simulink model "Tricopter_Controlled"  (R2015a)
settings: Solver=ode3  SolverMode=SingleTasking  StartTime=0.0  StopTime=inf  FixedStep=T_sim  RelTol=1e-3
values from neighbouring files (symbols this model uses):
  A_l_max_x = sqrt( (A_z_max)^2  -  g^2  )    [Run3Copter.m]
  A_l_max_y = g*tand(15)    [Run3Copter.m]
  A_z_max = Max_Thrust*3/m    [Run3Copter.m]
  Alt_0 = input(' Give the initial altitude (m): ')    [Run3Copter.m]
  B_hover_4dof = [-0.192641491537 -0.295051706147 -72.3190840892 -0.00308714144823 24.9504828653 -1.18743631629 9.87469464114e-05 6.48783896558 -0.0529805907426 -0.000387203135788 0.131620058452 2.24065603044 ... (54 elements, 6x9)]    [Effectiv_matrices.mat]
  CG_0 = [0,0,0.02]'    [SetupComplete.m]
  epsilon = 0.01    [Run3Copter.m]
  eta_23 = deg2rad(-1.3)    [Run3Copter.m]
  g = 9.81    [SetupComplete.m]
  h = 0.08    [SetupComplete.m]
  h_M = 0.064    [SetupComplete.m]
  Hover_eta_23 = deg2rad(-1.3)    [Run3Copter.m]
  Hover_throtle_1 = 0.745    [Run3Copter.m]
  Hover_throtle_23 = Hover_throtle_1/cos(Hover_eta_23)    [Run3Copter.m]
  I_BAC_0 = [ Ix,0,Ixz;0,Iy,0;Ixz,0,Iz]    [SetupComplete.m]
  Initial_Omegas = Omega_hover    [Run3Copter.m]
  Initial_Torques = Torque_hover    [Run3Copter.m]
  Ix = 0.103    [SetupComplete.m]
  Iy = 0.147    [SetupComplete.m]
  Iz = 0.237    [SetupComplete.m]
  l = 0.345    [SetupComplete.m]
  l_arm = 0.264    [SetupComplete.m]
  latitude = 52.071118    [Run3Copter.m]
  longitude = -0.627404    [Run3Copter.m]
  m = 3.51    [SetupComplete.m]
  m_0 = 2.61    [SetupComplete.m]
  m_M = 0.300    (= 0.3)    [SetupComplete.m]
  Rotation_sign = [ 1,-1,-1]    [SetupComplete.m]
  T_ctrl = 0.02    [Run3Copter.m]
  T_sim = 0.01    [Run3Copter.m]
  throtle_1 = 0*0.745    (= 0)    [Run3Copter.m]
  throtle_23 = throtle_1/cos(eta_23)    [Run3Copter.m]
  v_i0 = sqrt( 1/3*m*g/(2*rho*pi*R^2)  )    [SetupComplete.m]
undefined symbols (not defined in the file or in its folder): DOWN_0, EAST_0, Newton, NORTH_0, P_0, Q_0, R_0, Raphson, U_0, V_0, W_0
libraries: XXCopter_Control x64, simulink_extras x17, simulink x11, XXCopter x8
(part 5 of 6)

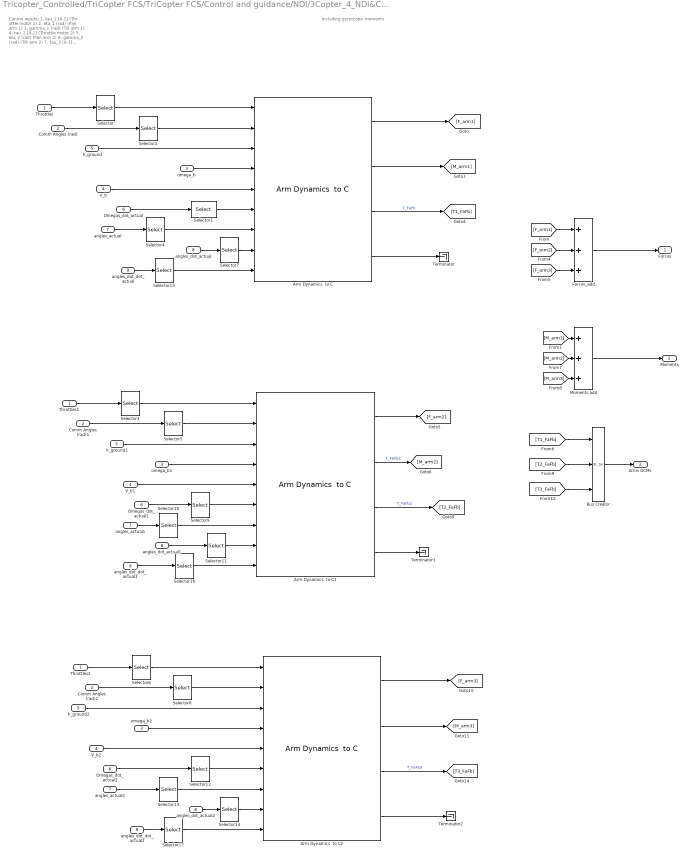
== system Tricopter_Controlled/TriCopter FCS/TriCopter FCS/Control and guidance/NDI/3Copter_4_NDI&CA/Arms Dynamics: Forces and Moments ==
  note: Including gyroscopic moments
  note: Control inputs:
      | 1. tau_1 [0-1] (Thr ottle motor 1)
      | 2. eta_1 (rad)  (Pan arm 1)
      | 3. gamma_1 (rad)  (Tilt arm 1)
      |
      | 4. tau_2 [0-1] (Throttle motor 2)
      | 5. eta_2 (rad)  (Pan arm 2)
      | 6. gamma_2 (rad)  (Tilt arm 2)
      |
      | 7. tau_3 [0-1] (Throttle motor 3)
      | 8. eta_3 (rad)  (Pan arm  3)
      | 9. gamma_3 (rad)  (Tilt arm 3)
  Throttles : Inport
  Comm Angles (rad) : Inport  Port=2
  omega_b : Inport  Port=3
  V_b : Inport  Port=4
  h_ground : Inport  Port=5
  Omegas_dot_actual : Inport  Port=6
  angles_actual : Inport  Port=7
  angles_dot_actual : Inport  Port=8
  angles_dot_dot_actual : Inport  Port=9
  Arm Dynamics  to C : XXCopter_Control/Arm Dynamics  to C  Rot_sign=Rotation_sign(1)  arm_hub_pos=l*[1;0;0]  Arm_axis=[l_arm;0;0]  arm_num=1  eta_dir=[1;0;0]  gamma_dir=[0;1;0]  J_T=J_T  J_FA=J_FA  h=h  switch_val=direct_feedforward  omega_n=30  xi=1.4  eta_inf_lim=deg2rad(-180)  eta_sup_lim=deg2rad(180)  gamma_inf_lim=deg2rad(-90)  gamma_sup_lim=deg2rad(15)
  Arm Dynamics  to C1 : XXCopter_Control/Arm Dynamics  to C  Rot_sign=Rotation_sign(2)  arm_hub_pos=l*[-1/2;sqrt(3)/2;0]  Arm_axis=[0;l_arm;0]  arm_num=2  eta_dir=[0;1;0]  gamma_dir=[1;0;0]  J_T=J_T  J_FA=J_FA  h=h  switch_val=direct_feedforward  omega_n=30  xi=1.4  eta_inf_lim=deg2rad(-180)  eta_sup_lim=deg2rad(180)  gamma_inf_lim=deg2rad(-15)  gamma_sup_lim=deg2rad(90)
  Arm Dynamics  to C2 : XXCopter_Control/Arm Dynamics  to C  Rot_sign=Rotation_sign(3)  arm_hub_pos=l*[-1/2;-sqrt(3)/2;0]  Arm_axis=[0;-l_arm;0]  arm_num=3  eta_dir=[0;1;0]  gamma_dir=[1;0;0]  J_T=J_T  J_FA=J_FA  h=h  switch_val=direct_feedforward  omega_n=30  xi=1.4  eta_inf_lim=deg2rad(-180)  eta_sup_lim=deg2rad(180)  gamma_inf_lim=deg2rad(-90)  gamma_sup_lim=deg2rad(15)
  Bus Creator : BusCreator  Inputs=3
  Comm Angles (rad)1 : InportShadow  Port=2
  Comm Angles (rad)2 : InportShadow  Port=2
  Forces_add : Sum  Inputs=+++
  Moments add : Sum  Inputs=+++
  Omegas_dot_actual1 : InportShadow  Port=6
  Omegas_dot_actual2 : InportShadow  Port=6
  Selector : Selector  IndexMode=Zero-based  InputPortWidth=3  Indices=0
  Selector1 : Selector  IndexMode=Zero-based  InputPortWidth=3  Indices=0
  Selector{5,10..11,16} (4 alike) : Selector  IndexMode=Zero-based  InputPortWidth=6  Indices=[2,3]
  Selector12 : Selector  IndexMode=Zero-based  InputPortWidth=3  Indices=2
  Selector{8,13..14,17} (4 alike) : Selector  IndexMode=Zero-based  InputPortWidth=6  Indices=[4,5]
  Selector{2,4,7,15} (4 alike) : Selector  IndexMode=Zero-based  InputPortWidth=6  Indices=[0,1]
  Selector3 : Selector  IndexMode=Zero-based  InputPortWidth=3
  Selector6 : Selector  IndexMode=Zero-based  InputPortWidth=3  Indices=2
  Selector9 : Selector  IndexMode=Zero-based  InputPortWidth=3
  Terminator : Terminator
  Terminator1 : Terminator
  Terminator2 : Terminator
  Throttles1 : InportShadow
  Throttles2 : InportShadow
  V_b1 : InportShadow  Port=4
  V_b2 : InportShadow  Port=4
  angles_actual1 : InportShadow  Port=7
  angles_actual2 : InportShadow  Port=7
  angles_dot_actual1 : InportShadow  Port=8
  angles_dot_actual2 : InportShadow  Port=8
  angles_dot_dot_actual1 : InportShadow  Port=9
  angles_dot_dot_actual2 : InportShadow  Port=9
  h_ground1 : InportShadow  Port=5
  h_ground2 : InportShadow  Port=5
  omega_b1 : InportShadow  Port=3
  omega_b2 : InportShadow  Port=3
  Forces : Outport
  Moments : Outport  Port=2
  Arms DCMs : Outport  Port=3
  wires:
  Selector14/1 -> Arm Dynamics  to C2/8
  angles_actual2/1 -> Selector13/1
  angles_dot_actual2/1 -> Selector14/1
  Selector13/1 -> Arm Dynamics  to C2/7
  Selector12/1 -> Arm Dynamics  to C2/6
  Omegas_dot_actual2/1 -> Selector12/1
  Selector11/1 -> Arm Dynamics  to C1/8
  angles_actual1/1 -> Selector10/1
  angles_dot_actual1/1 -> Selector11/1
  Selector10/1 -> Arm Dynamics  to C1/7
  Selector9/1 -> Arm Dynamics  to C1/6
  Omegas_dot_actual1/1 -> Selector9/1
  Selector7/1 -> Arm Dynamics  to C/8
  angles_dot_actual/1 -> Selector7/1
  Selector4/1 -> Arm Dynamics  to C/7
  angles_actual/1 -> Selector4/1
  Selector1/1 -> Arm Dynamics  to C/6
  Omegas_dot_actual/1 -> Selector1/1
  [T3_FaFb] -> Bus Creator/3
  [T2_FaFb] -> Bus Creator/2
  [T1_FaFb] -> Bus Creator/1
  Bus Creator/1 -> Arms DCMs/1
  Arm Dynamics  to C1/2 -> [M_arm2]  "T_FaFb2"
  Arm Dynamics  to C1/1 -> [F_arm2]
  Arm Dynamics  to C2/4 -> Terminator2/1
  Arm Dynamics  to C1/4 -> Terminator1/1
  Arm Dynamics  to C/4 -> Terminator/1
  Arm Dynamics  to C2/3 -> [T3_FaFb]  "T_FaFb3"
  Comm Angles (rad)2/1 -> Selector8/1
  Selector8/1 -> Arm Dynamics  to C2/2
  omega_b2/1 -> Arm Dynamics  to C2/4
  Arm Dynamics  to C2/2 -> [M_arm3]
  Arm Dynamics  to C2/1 -> [F_arm3]
  h_ground2/1 -> Arm Dynamics  to C2/3
  V_b2/1 -> Arm Dynamics  to C2/5
  Selector6/1 -> Arm Dynamics  to C2/1
  Throttles2/1 -> Selector6/1
  Arm Dynamics  to C1/3 -> [T2_FaFb]  "T_FaFb2"
  Comm Angles (rad)1/1 -> Selector5/1
  Selector5/1 -> Arm Dynamics  to C1/2
  omega_b1/1 -> Arm Dynamics  to C1/4
  h_ground1/1 -> Arm Dynamics  to C1/3
  V_b1/1 -> Arm Dynamics  to C1/5
  Selector3/1 -> Arm Dynamics  to C1/1
  Throttles1/1 -> Selector3/1
  Arm Dynamics  to C/3 -> [T1_FaFb]  "T_FaFb"
  Comm Angles (rad)/1 -> Selector2/1
  Selector2/1 -> Arm Dynamics  to C/2
  [M_arm2] -> Moments add/2
  [M_arm3] -> Moments add/3
  [F_arm3] -> Forces_add/3
  [F_arm2] -> Forces_add/2
  omega_b/1 -> Arm Dynamics  to C/4
  [M_arm1] -> Moments add/1
  [F_arm1] -> Forces_add/1
  Arm Dynamics  to C/2 -> [M_arm1]
  Arm Dynamics  to C/1 -> [F_arm1]
  h_ground/1 -> Arm Dynamics  to C/3
  Moments add/1 -> Moments/1
  Forces_add/1 -> Forces/1
  V_b/1 -> Arm Dynamics  to C/5
  Selector/1 -> Arm Dynamics  to C/1
  Throttles/1 -> Selector/1
  angles_dot_dot_actual/1 -> Selector15/1
  Selector15/1 -> Arm Dynamics  to C/9
  angles_dot_dot_actual1/1 -> Selector16/1
  Selector16/1 -> Arm Dynamics  to C1/9
  angles_dot_dot_actual2/1 -> Selector17/1
  Selector17/1 -> Arm Dynamics  to C2/9

== system Tricopter_Controlled/TriCopter FCS/TriCopter FCS/Control and guidance/NDI/3Copter_4_NDI&CA/Gradient ==
  note: Control inputs:
      | 1. tau_1 [0-1] (Thr ottle motor 1)
      | 2. eta_1 (rad)  (Pan arm 1)
      | 3. gamma_1 (rad)  (Tilt arm 1)
      |
      | 4. tau_2 [0-1] (Throttle motor 2)
      | 5. eta_2 (rad)  (Pan arm 2)
      | 6. gamma_2 (rad)  (Tilt arm 2)
      |
      | 7. tau_3 [0-1] (Throttle motor 3)
      | 8. eta_3 (rad)  (Pan arm  3)
      | 9. gamma_3 (rad)  (Tilt arm 3)
  Curr_V : Inport  Partition=off
  "Control Inputs(rad) " : Inport  Port=2  Partition=on  PartitionDimension=1  PartitionWidth=9
  h : Inport  Port=3  Partition=off
  Vb : Inport  Port=4  Partition=off
  omega_b : Inport  Port=5  Partition=off
  Omegas_dot_actual : Inport  Port=6  Partition=off
  angles_actual : Inport  Port=7  Partition=off
  angles_dot_actual : Inport  Port=8  Partition=off
  angles_dot_dot_actual : Inport  Port=9  Partition=off
  F_g : Inport  Port=10  Partition=off
  M_g : Inport  Port=11  Partition=off
  Add : Sum
  Add1 : Sum
  Arms Dynamics: Forces and Moments : Subsystem  TreatAsAtomicUnit=on
  Equivalent Throttle : Product  Inputs=**
  For Each : ForEach  DisableCoverage=on  IndexMode=One-based
  Mux : Mux  Inputs=[3,3]
  Signal Specification : SignalSpecification  Dimensions=[6,1]
  Terminator : Terminator
  Throttles : Selector  IndexMode=Zero-based  InputPortWidth=9  Indices=[0,3,6]
  "angles " : Selector  IndexMode=Zero-based  InputPortWidth=9  Indices=[1,2,4,5,7,8]
  Forces_Moments : Outport  ConcatenationDimension=2
  wires:
  Signal Specification/1 -> Forces_Moments/1
  Mux/1 -> Signal Specification/1
  Add1/1 -> Mux/2
  Add/1 -> Mux/1
  M_g/1 -> Add1/2
  F_g/1 -> Add/2
  angles_dot_actual/1 -> Arms Dynamics: Forces and Moments/8(angles_dot_actual)
  Omegas_dot_actual/1 -> Arms Dynamics: Forces and Moments/6(Omegas_dot_actual)
  Curr_V/1 -> Equivalent Throttle/1
  Equivalent Throttle/1 -> Arms Dynamics: Forces and Moments/1(Throttles)
  "Control Inputs(rad) "/1 -> "angles "/1, Throttles/1
  Throttles/1 -> Equivalent Throttle/2
  Arms Dynamics: Forces and Moments/1(Forces) -> Add/1
  h/1 -> Arms Dynamics: Forces and Moments/5(h_ground)
  omega_b/1 -> Arms Dynamics: Forces and Moments/3(omega_b)
  angles_actual/1 -> Arms Dynamics: Forces and Moments/7(angles_actual)
  "angles "/1 -> Arms Dynamics: Forces and Moments/2(Comm Angles (rad))
  angles_dot_dot_actual/1 -> Arms Dynamics: Forces and Moments/9(angles_dot_dot_actual)
  Arms Dynamics: Forces and Moments/2(Moments) -> Add1/1
  Arms Dynamics: Forces and Moments/3(Arms DCMs) -> Terminator/1
  Vb/1 -> Arms Dynamics: Forces and Moments/4(V_b)

== system Tricopter_Controlled/TriCopter FCS/TriCopter FCS/Control and guidance/NDI/3Copter_4_NDI&CA/Ground  model ==
  h : Inport
  m : Inport  Port=2
  q : Inport  Port=3
  Ground model logic and Forces and moments : MATLAB Function  TreatAsAtomicUnit=on
  arm_hub position 1 : Constant  Value=l*[1;0;0]
  arm_hub position 2 : Constant  Value=l*[-1/2;sqrt(3)/2;0]
  arm_hub position 3 : Constant  Value=l*[-1/2;-sqrt(3)/2;0]
  F_ground : Outport
  wires:
  h/1 -> Ground model logic and Forces and moments/1(h)
  m/1 -> Ground model logic and Forces and moments/2(mass)
  arm_hub position 1/1 -> Ground model logic and Forces and moments/4(Arm1)
  arm_hub position 2/1 -> Ground model logic and Forces and moments/5(Arm2)
  arm_hub position 3/1 -> Ground model logic and Forces and moments/6(Arm3)
  Ground model logic and Forces and moments/1(F_gr_b) -> F_ground/1
  q/1 -> Ground model logic and Forces and moments/3(q)

== system Tricopter_Controlled/TriCopter FCS/TriCopter FCS/Control and guidance/NDI/3Copter_4_NDI&CA/Mass Properties ==
  Arms DCMs : Inport
  CG_0 : Inport  Port=2
  m_0 : Inport  Port=3
  m : Inport  Port=4
  m_M : Inport  Port=5
  I_BAC_0 : Inport  Port=6
  Arm Inertia : MATLAB Function  TreatAsAtomicUnit=on
  Bus Selector : BusSelector  OutputSignals=T_FaFb,T_FaFb2,T_FaFb3
  CG position : Sum
  Divide : Product  Inputs=*/
  Divide1 : Product  Inputs=**
  Divide2 : Product  Inputs=/*
  Divide3 : Product  Inputs=**
  Motors Pos sum : Sum  Inputs=+++
  Total I_BAC : Sum
  I_BAC : Outport
  CG : Outport  Port=2
  wires:
  Arm Inertia/2(r1_M) -> Motors Pos sum/3
  I_BAC_0/1 -> Total I_BAC/1
  Arm Inertia/1(I_M) -> Total I_BAC/2
  Arm Inertia/4(r3_M) -> Motors Pos sum/1
  Arm Inertia/3(r2_M) -> Motors Pos sum/2
  Divide3/1 -> CG position/2
  Divide2/1 -> Divide3/2
  Motors Pos sum/1 -> Divide3/1
  Divide1/1 -> CG position/1
  CG position/1 -> CG/1
  m_M/1 -> Divide2/2
  Divide/1 -> Divide1/2
  CG_0/1 -> Divide1/1
  m/1 -> Divide2/1, Divide/2
  m_0/1 -> Divide/1
  Total I_BAC/1 -> I_BAC/1
  Bus Selector/1 -> Arm Inertia/1(T1_FAFb)  "<T_FaFb>"
  Bus Selector/2 -> Arm Inertia/2(T2_FAFb)  "<T_FaFb2>"
  Bus Selector/3 -> Arm Inertia/3(T3_FAFb)  "<T_FaFb3>"
  Arms DCMs/1 -> Bus Selector/1

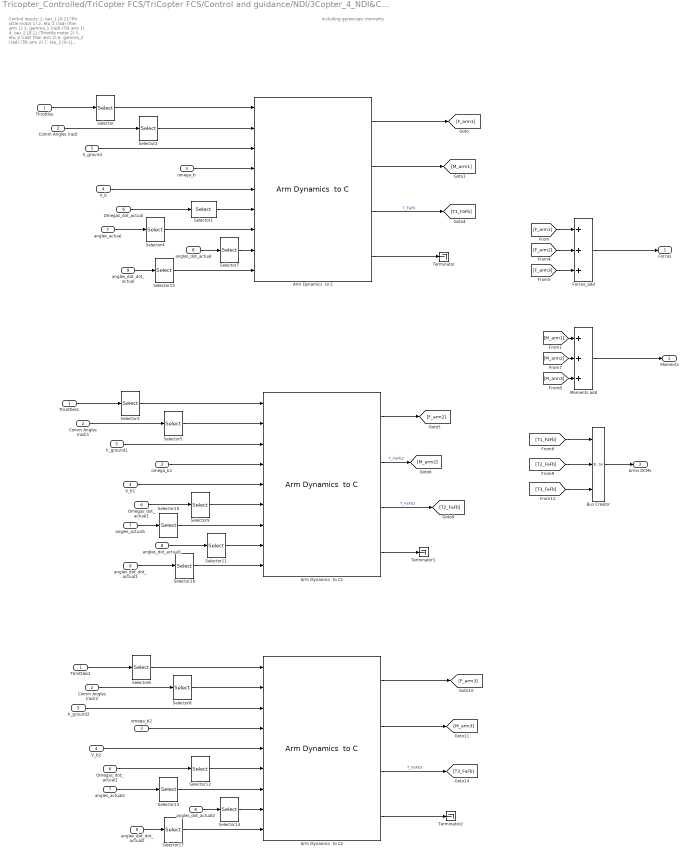
== system Tricopter_Controlled/TriCopter FCS/TriCopter FCS/Control and guidance/NDI/3Copter_4_NDI&CA/Gradient/Arms Dynamics: Forces and Moments ==
  note: Including gyroscopic moments
  note: Control inputs:
      | 1. tau_1 [0-1] (Thr ottle motor 1)
      | 2. eta_1 (rad)  (Pan arm 1)
      | 3. gamma_1 (rad)  (Tilt arm 1)
      |
      | 4. tau_2 [0-1] (Throttle motor 2)
      | 5. eta_2 (rad)  (Pan arm 2)
      | 6. gamma_2 (rad)  (Tilt arm 2)
      |
      | 7. tau_3 [0-1] (Throttle motor 3)
      | 8. eta_3 (rad)  (Pan arm  3)
      | 9. gamma_3 (rad)  (Tilt arm 3)
  Throttles : Inport
  Comm Angles (rad) : Inport  Port=2
  omega_b : Inport  Port=3
  V_b : Inport  Port=4
  h_ground : Inport  Port=5
  Omegas_dot_actual : Inport  Port=6
  angles_actual : Inport  Port=7
  angles_dot_actual : Inport  Port=8
  angles_dot_dot_actual : Inport  Port=9
  Arm Dynamics  to C : XXCopter_Control/Arm Dynamics  to C  Rot_sign=Rotation_sign(1)  arm_hub_pos=l*[1;0;0]  Arm_axis=[l_arm;0;0]  arm_num=1  eta_dir=[1;0;0]  gamma_dir=[0;1;0]  J_T=J_T  J_FA=J_FA  h=h  switch_val=direct_feedforward  omega_n=30  xi=1.4  eta_inf_lim=deg2rad(-180)  eta_sup_lim=deg2rad(180)  gamma_inf_lim=deg2rad(-90)  gamma_sup_lim=deg2rad(15)
  Arm Dynamics  to C1 : XXCopter_Control/Arm Dynamics  to C  Rot_sign=Rotation_sign(2)  arm_hub_pos=l*[-1/2;sqrt(3)/2;0]  Arm_axis=[0;l_arm;0]  arm_num=2  eta_dir=[0;1;0]  gamma_dir=[1;0;0]  J_T=J_T  J_FA=J_FA  h=h  switch_val=direct_feedforward  omega_n=30  xi=1.4  eta_inf_lim=deg2rad(-180)  eta_sup_lim=deg2rad(180)  gamma_inf_lim=deg2rad(-15)  gamma_sup_lim=deg2rad(90)
  Arm Dynamics  to C2 : XXCopter_Control/Arm Dynamics  to C  Rot_sign=Rotation_sign(3)  arm_hub_pos=l*[-1/2;-sqrt(3)/2;0]  Arm_axis=[0;-l_arm;0]  arm_num=3  eta_dir=[0;1;0]  gamma_dir=[1;0;0]  J_T=J_T  J_FA=J_FA  h=h  switch_val=direct_feedforward  omega_n=30  xi=1.4  eta_inf_lim=deg2rad(-180)  eta_sup_lim=deg2rad(180)  gamma_inf_lim=deg2rad(-90)  gamma_sup_lim=deg2rad(15)
  Bus Creator : BusCreator  Inputs=3
  Comm Angles (rad)1 : InportShadow  Port=2
  Comm Angles (rad)2 : InportShadow  Port=2
  Forces_add : Sum  Inputs=+++
  Moments add : Sum  Inputs=+++
  Omegas_dot_actual1 : InportShadow  Port=6
  Omegas_dot_actual2 : InportShadow  Port=6
  Selector : Selector  IndexMode=Zero-based  InputPortWidth=3  Indices=0
  Selector1 : Selector  IndexMode=Zero-based  InputPortWidth=3  Indices=0
  Selector{5,10..11,16} (4 alike) : Selector  IndexMode=Zero-based  InputPortWidth=6  Indices=[2,3]
  Selector12 : Selector  IndexMode=Zero-based  InputPortWidth=3  Indices=2
  Selector{8,13..14,17} (4 alike) : Selector  IndexMode=Zero-based  InputPortWidth=6  Indices=[4,5]
  Selector{2,4,7,15} (4 alike) : Selector  IndexMode=Zero-based  InputPortWidth=6  Indices=[0,1]
  Selector3 : Selector  IndexMode=Zero-based  InputPortWidth=3
  Selector6 : Selector  IndexMode=Zero-based  InputPortWidth=3  Indices=2
  Selector9 : Selector  IndexMode=Zero-based  InputPortWidth=3
  Terminator : Terminator
  Terminator1 : Terminator
  Terminator2 : Terminator
  Throttles1 : InportShadow
  Throttles2 : InportShadow
  V_b1 : InportShadow  Port=4
  V_b2 : InportShadow  Port=4
  angles_actual1 : InportShadow  Port=7
  angles_actual2 : InportShadow  Port=7
  angles_dot_actual1 : InportShadow  Port=8
  angles_dot_actual2 : InportShadow  Port=8
  angles_dot_dot_actual1 : InportShadow  Port=9
  angles_dot_dot_actual2 : InportShadow  Port=9
  h_ground1 : InportShadow  Port=5
  h_ground2 : InportShadow  Port=5
  omega_b1 : InportShadow  Port=3
  omega_b2 : InportShadow  Port=3
  Forces : Outport
  Moments : Outport  Port=2
  Arms DCMs : Outport  Port=3
  wires:
  Selector14/1 -> Arm Dynamics  to C2/8
  angles_actual2/1 -> Selector13/1
  angles_dot_actual2/1 -> Selector14/1
  Selector13/1 -> Arm Dynamics  to C2/7
  Selector12/1 -> Arm Dynamics  to C2/6
  Omegas_dot_actual2/1 -> Selector12/1
  Selector11/1 -> Arm Dynamics  to C1/8
  angles_actual1/1 -> Selector10/1
  angles_dot_actual1/1 -> Selector11/1
  Selector10/1 -> Arm Dynamics  to C1/7
  Selector9/1 -> Arm Dynamics  to C1/6
  Omegas_dot_actual1/1 -> Selector9/1
  Selector7/1 -> Arm Dynamics  to C/8
  angles_dot_actual/1 -> Selector7/1
  Selector4/1 -> Arm Dynamics  to C/7
  angles_actual/1 -> Selector4/1
  Selector1/1 -> Arm Dynamics  to C/6
  Omegas_dot_actual/1 -> Selector1/1
  [T3_FaFb] -> Bus Creator/3
  [T2_FaFb] -> Bus Creator/2
  [T1_FaFb] -> Bus Creator/1
  Bus Creator/1 -> Arms DCMs/1
  Arm Dynamics  to C1/2 -> [M_arm2]  "T_FaFb2"
  Arm Dynamics  to C1/1 -> [F_arm2]
  Arm Dynamics  to C2/4 -> Terminator2/1
  Arm Dynamics  to C1/4 -> Terminator1/1
  Arm Dynamics  to C/4 -> Terminator/1
  Arm Dynamics  to C2/3 -> [T3_FaFb]  "T_FaFb3"
  Comm Angles (rad)2/1 -> Selector8/1
  Selector8/1 -> Arm Dynamics  to C2/2
  omega_b2/1 -> Arm Dynamics  to C2/4
  Arm Dynamics  to C2/2 -> [M_arm3]
  Arm Dynamics  to C2/1 -> [F_arm3]
  h_ground2/1 -> Arm Dynamics  to C2/3
  V_b2/1 -> Arm Dynamics  to C2/5
  Selector6/1 -> Arm Dynamics  to C2/1
  Throttles2/1 -> Selector6/1
  Arm Dynamics  to C1/3 -> [T2_FaFb]  "T_FaFb2"
  Comm Angles (rad)1/1 -> Selector5/1
  Selector5/1 -> Arm Dynamics  to C1/2
  omega_b1/1 -> Arm Dynamics  to C1/4
  h_ground1/1 -> Arm Dynamics  to C1/3
  V_b1/1 -> Arm Dynamics  to C1/5
  Selector3/1 -> Arm Dynamics  to C1/1
  Throttles1/1 -> Selector3/1
  Arm Dynamics  to C/3 -> [T1_FaFb]  "T_FaFb"
  Comm Angles (rad)/1 -> Selector2/1
  Selector2/1 -> Arm Dynamics  to C/2
  [M_arm2] -> Moments add/2
  [M_arm3] -> Moments add/3
  [F_arm3] -> Forces_add/3
  [F_arm2] -> Forces_add/2
  omega_b/1 -> Arm Dynamics  to C/4
  [M_arm1] -> Moments add/1
  [F_arm1] -> Forces_add/1
  Arm Dynamics  to C/2 -> [M_arm1]
  Arm Dynamics  to C/1 -> [F_arm1]
  h_ground/1 -> Arm Dynamics  to C/3
  Moments add/1 -> Moments/1
  Forces_add/1 -> Forces/1
  V_b/1 -> Arm Dynamics  to C/5
  Selector/1 -> Arm Dynamics  to C/1
  Throttles/1 -> Selector/1
  angles_dot_dot_actual/1 -> Selector15/1
  Selector15/1 -> Arm Dynamics  to C/9
  angles_dot_dot_actual1/1 -> Selector16/1
  Selector16/1 -> Arm Dynamics  to C1/9
  angles_dot_dot_actual2/1 -> Selector17/1
  Selector17/1 -> Arm Dynamics  to C2/9

== matlab function Tricopter_Controlled/3 Copter Complete/6dof Eqs of motion/Position Eqs ==
  data: A_b output; Vb input; omega input; omega_dot input; Forces input; m input; CG input
function A_b  = PositionEqs(Vb,omega,omega_dot, Forces,m, CG)



 
A_b =  1/m*( Forces ) - cross(omega,Vb) - cross(omega, cross(omega,CG)) -cross(omega_dot,CG)  ;

== matlab function Tricopter_Controlled/3 Copter Complete/6dof Eqs of motion/Rotational eqs ==
  data: omega_dot output; omega_b input; Moments input; I_BAC input
function omega_dot  = Rotational_Eq(omega_b,Moments, I_BAC)



omega_dot =  I_BAC\( Moments - cross(omega_b,I_BAC*omega_b)  );

== matlab function Tricopter_Controlled/3 Copter Complete/6dof Eqs of motion/q_dot/Quaternion_dot ==
  data: omega_b input; q_dot output; q input
function q_dot = Quaternion_dot(omega_b,q)


q_dot = 1/2*HamiltonProduct(q,[0;omega_b]);

function Product= HamiltonProduct( a,b )

Product=[ a(1)*b(1)-a(2)*b(2)-a(3)*b(3)-a(4)*b(4) ; a(1)*b(2)+a(2)*b(1)+a(3)*b(4)-a(4)*b(3)  ; a(1)*b(3)-a(2)*b(4)+a(3)*b(1)+a(4)*b(2)  ; a(1)*b(4)+a(2)*b(3)-a(3)*b(2)+a(4)*b(1) ];

== matlab function Tricopter_Controlled/TriCopter FCS/TriCopter FCS/Flight mode manager and commands generator/Flight manager/Parameters_based_decision_making ==
  data: flight_mode_out output; flight_mode input; pdop input; vdop input; num_sats input; Alt input; Volt input; Accs input
function flight_mode_out     =  Params_decision_making(flight_mode,pdop,vdop,num_sats,Alt,Volt,Accs)

% si esta en landing y recive una aceleracion vertical de <-5m/s^2( Hacia
% arriba), pasar a modo OFF

% If ready from off blue LED
flight_mode_out = flight_mode;
 switch flight_mode % Being in this FM
        case 0 % Off
           
        case 1 % Ready
         
        case 2 % Take off
           
        case 3 % Full_auto
           
        case 4 % Vel_height_auto
           
        case 5 % Vel_auto
           
        case 6 % Stab
           
        case 7 % Man_ctrl
            
        case 8 % Home
            
        case 9 % Land
          
        otherwise
            flight_mode_out = flight_mode;
 end

== matlab function Tricopter_Controlled/TriCopter FCS/TriCopter FCS/Control and guidance/Inner PI Controller Quaternions/Attitude Controller/Build Pseudo_theta1 ==
  data: q input; Pseudo_theta output
function Pseudo_theta    = F_Pseudo_theta( q)


%% Actitud en Angulos de Euler y sus derivadas.
Pseudo_theta=0;
Pseudo_theta = ( 2*q(2)*q(4)-2*q(1)*q(3) ); %  pseudo-theta




end

== matlab function Tricopter_Controlled/TriCopter FCS/TriCopter FCS/flight_mode_effector/flight_mode_effector ==
  data: flight_mode input; pos_xy_act output boolean; alt_act output boolean; vel_yaw_xy_act output boolean; vel_yaw_z_act output boolean; att_act output boolean; omega_b_act output boolean; pos_xy_init output; alt_init output; vel_yaw_xy_init output; vel_yaw_z_init output; att_init output; b_rates_init output; X_e input; CA_reconf output; V_yaw input; Euler input; omega_b input; Armed output
function [pos_xy_act,alt_act,vel_yaw_xy_act,vel_yaw_z_act,att_act,omega_b_act,pos_xy_init,alt_init,vel_yaw_xy_init,vel_yaw_z_init,att_init,b_rates_init,CA_reconf,Armed]   =  flight_mode_effector(flight_mode,X_e,V_yaw,Euler, omega_b)
%% Efector de los modos de vuelos
% Hace efectivos los cambios en los modos de vuelo en el controlador

%% CA_reconf
% CA_reconf = 1 : Control in 9dof with Incremental CA
% CA_reconf = 2 :  Control in 4dof with NO Incremental CA. Assumed to be a "safe" mode

%% Armed
% Armed = 0 No armed
% Armed = 1 Armed

%% Activate vectors
% 0 means no activated
% 1 means activated


switch flight_mode
    case 0 % Off
        pos_xy_act      = false;     
        alt_act         = false;
        vel_yaw_xy_act  = false; 
        vel_yaw_z_act   = false; 
        att_act         = false;
        omega_b_act     = false;
        
        pos_xy_init     = [0;0];     
        alt_init        = 0;
        vel_yaw_xy_init = [0;0]; 
        vel_yaw_z_init  = 0;
        att_init        = [0;0;0]; 
        b_rates_init    = [0;0;0];
        
        CA_reconf = 2;
        
        Armed = 0;
    case 1 % Ready
        pos_xy_act      = false;     
        alt_act         = false;
        vel_yaw_xy_act  = false; 
        vel_yaw_z_act   = false; 
        att_act         = false; 
        omega_b_act     = false;
        
        pos_xy_init     = [0;0];     
        alt_init        = 0;
        vel_yaw_xy_init = [0;0]; 
        vel_yaw_z_init  = 0;
        att_init        = [0;0;0]; 
        b_rates_init    = [0;0;0];
        
        CA_reconf = 2;
        
        Armed = 0;
    case 2 % Take off
        pos_xy_act      = true;     
        alt_act         = true;
        vel_yaw_xy_act  = true; 
        vel_yaw_z_act   = true; 
        att_act         = true; 
        omega_b_act     = true;
        
        pos_xy_init     = [0;0];    
        alt_init        = X_e(3);     
        vel_yaw_xy_init = [0;0]; 
        vel_yaw_z_init  = 0;
        att_init        = [0;0;Euler(3)]; 
        b_rates_init    = [0;0;0];
        
        CA_reconf = 1;
        
        Armed = 1;
    case 3 % Full_auto
        pos_xy_act      = true;     
        alt_act         = true;
        vel_yaw_xy_act  = true; 
        vel_yaw_z_act   = true; 
        att_act         = true; 
        omega_b_act     = true;
        
        pos_xy_init     = X_e(1:2);    
        alt_init        = X_e(3);     
        vel_yaw_xy_init = [V_yaw(1);V_yaw(2)]; 
        vel_yaw_z_init  = V_yaw(3);
        att_init        = [Euler(1);Euler(2);Euler(3)]; 
        b_rates_init    = omega_b;
        
        CA_reconf = 1;
        
        Armed = 1;
    case 4 % Vel_height_auto
        pos_xy_act      = false;     
        alt_act         = true;
        vel_yaw_xy_act  = true; 
        vel_yaw_z_act   = true; 
        att_act         = true; 
        omega_b_act     = true;
        
        pos_xy_init     = [0;0];    
        alt_init        = X_e(3);      
        vel_yaw_xy_init = [V_yaw(1);V_yaw(2)]; 
        vel_yaw_z_init  = V_yaw(3);
        att_init        = [Euler(1);Euler(2);Euler(3)]; 
        b_rates_init    = omega_b;
        
        CA_reconf = 1;
        
        Armed = 1;
    case 5 % Vel_auto
        pos_xy_act      = false;     
        alt_act         = false;
        vel_yaw_xy_act  = true; 
        vel_yaw_z_act   = true; 
        att_act         = true; 
        omega_b_act     = true;
        
        pos_xy_init     = [0;0];    
        alt_init        = 0;      
        vel_yaw_xy_init = [V_yaw(1);V_yaw(2)]; 
        vel_yaw_z_init  = V_yaw(3);
        att_init        = [Euler(1);Euler(2);Euler(3)]; 
        b_rates_init    = omega_b;
        
        CA_reconf = 1;
        
        Armed = 1;
    case 6 % Stab
        pos_xy_act      = false;     
        alt_act         = false;
        vel_yaw_xy_act  = false; 
        vel_yaw_z_act   = true; 
        att_act         = true; 
        omega_b_act     = true;
        
        pos_xy_init     = [0;0];    
        alt_init        = 0;     
        vel_yaw_xy_init = [0;0]; 
        vel_yaw_z_init  = 0;
        att_init        = [Euler(1);Euler(2);Euler(3)]; 
        b_rates_init    = omega_b;
        
        CA_reconf = 2;
        
        Armed = 1;
    case 7 % Man_ctrl
        pos_xy_act      = false;     
        alt_act         = false;
        vel_yaw_xy_act  = false; 
        vel_yaw_z_act   = true; 
        att_act         = false; 
        omega_b_act     = true;
        
        pos_xy_init     = [0;0];    
        alt_init        = 0;      
        vel_yaw_xy_init = [0;0]; 
        vel_yaw_z_init  = 0;
        att_init        = [0;0;0]; 
        b_rates_init    = [0;0;0]; 
        
        CA_reconf = 2;
        
        Armed = 1;
    case 8 % Home
        pos_xy_act      = true;     
        alt_act         = true;
        vel_yaw_xy_act  = true; 
        vel_yaw_z_act   = true; 
        att_act         = true; 
        omega_b_act     = true;
        
        pos_xy_init     = X_e(1:2);    
        alt_init        = X_e(3);      
        vel_yaw_xy_init = [V_yaw(1);V_yaw(2)]; 
        vel_yaw_z_init  = V_yaw(3);
        att_init        = [Euler(1);Euler(2);Euler(3)]; 
        b_rates_init    = omega_b; 
        
        CA_reconf = 1;
        
        Armed = 1;
        
    case 9 % Land
        pos_xy_act      = true;     
        alt_act         = true;
        vel_yaw_xy_act  = true; 
        vel_yaw_z_act   = true; 
        att_act         = true; 
        omega_b_act     = true;
        
        pos_xy_init     = X_e(1:2);    
        alt_init        = X_e(3);      
        vel_yaw_xy_init = [V_yaw(1);V_yaw(2)];
        vel_yaw_z_init  = V_yaw(3);
        att_init        = [Euler(1);Euler(2);Euler(3)]; 
        b_rates_init    = omega_b;
        
        CA_reconf = 1;
        
        Armed = 1;
    otherwise
        pos_xy_act      = false;     
        alt_act         = false;
        vel_yaw_xy_act  = false; 
        vel_yaw_z_act   = false; 
        att_act         = false; 
        omega_b_act     = false;
        
        pos_xy_init     = [0;0];    
        alt_init        = 0;      
        vel_yaw_xy_init = [0;0]; 
        vel_yaw_z_init  = 0;
        att_init        = [0;0;0]; 
        b_rates_init    = [0;0;0]; 
        
        CA_reconf = 2;
        
        Armed = 0;
        
end

== matlab function Tricopter_Controlled/3 Copter Complete/6dof Eqs of motion/Eccelerometer meas ==
  data: Vb input; omega input; omega_dot input; Ab input; A_s output; r_sens parameter
function A_s  = AcellMeas(Vb,omega,omega_dot,Ab, r_sens)




A_s =  Ab + cross(omega,Vb) + cross(omega, cross(omega,r_sens)) +cross(omega_dot,r_sens)  ;

== matlab function Tricopter_Controlled/TriCopter FCS/TriCopter FCS/Control and guidance/Inner PI Controller Quaternions/MATLAB Function ==
  data: omega_b input size=[3,1]; Euler_dot output; Euler input size=[3,1]
function Euler_dot = omega2Euler_dot(omega_b,Euler)

phi = Euler(1);
theta = Euler(2);
psi = Euler(3);


A = [1          0               -sin(theta)         ;
     0          cos(phi)        sin(phi)*cos(theta) ;
     0          -sin(phi)       cos(phi)*cos(theta)];

Euler_dot = A'*omega_b ;

== matlab function Tricopter_Controlled/TriCopter FCS/TriCopter FCS/Control and guidance/NDI/3Copter_4_NDI&CA/Get gradient ==
  data: epsilon input; CA_Grad output; Perturb_evaluations input
function CA_Grad  = Get_gradient(epsilon,Perturb_evaluations)

CA_Grad = zeros(6,9);

for i=1:9
    CA_Grad(:,i)= ( Perturb_evaluations(:,2*i)-Perturb_evaluations(:,2*i-1)  )./(epsilon);
end

%% 4 DOF
% CA_Grad(:,3)=zeros(6,1);
% CA_Grad(:,5:6)=zeros(6,2);
% CA_Grad(:,8:9)=zeros(6,2);
% 

%% Just diff throtle
% CA_Grad(3:5,2:3)=zeros(3,2);
% CA_Grad(3:5,5:6)=zeros(3,2);
% CA_Grad(3:5,8:9)=zeros(3,2);


end

== matlab function Tricopter_Controlled/3 Copter Complete/6dof Eqs of motion/SVFI_to_SVFb ==
  data: X_e input; V_e input; X_e_out output; V_b output; omega_b output; Euler_Ang input; Euler_Ang_Dot input; q output
function [X_e_out,V_b, omega_b ,q]=SVFI_to_SVFb(X_e,V_e, Euler_Ang,Euler_Ang_Dot)

q = zeros(4,1);
V_b =zeros(3,1);

xp=V_e(1);
yp=V_e(2);
zp=V_e(3);

phi=Euler_Ang(1);
theta=Euler_Ang(2);
psi=Euler_Ang(3);
phip=Euler_Ang_Dot(1);
thetap=Euler_Ang_Dot(2);
psip=Euler_Ang_Dot(3);

%%
X_e_out=X_e;

q = QuaternionfromEuler(phi,theta,psi); 



HamOut=HamiltonProduct([q(1);-q(2);-q(3);-q(4)],HamiltonProduct([0;xp;yp;zp],[q(1);q(2);q(3);q(4)]) );% q* . v . q
V_b=HamOut(2:4);

omega_b=[phip-psip*sin(theta)  ;
         thetap*cos(phi)+psip*cos(theta)*sin(phi);
            -thetap*sin(phi)+psip*cos(theta)*cos(phi)  ];% Ya que es solo una operacion aislada utilizaremos la ecuaciones con rel trigonometricas

function [q]=QuaternionfromEuler(phi,theta,psi)
% options=optimset('MaxFunEvals',3000);
% q=fsolve(@QUATERNIONEULER,[0.6,0.4,0.5,0.4]); % Hay que acertar con los angulos poniendo diferentes valores iniciales del quaternion
%     function F=QUATERNIONEULER(q)
%         F=[ tan(phi)-(2*q(3)*q(4)-2*q(1)*q(2))/(2*q(1)^2+2*q(4)^2-1)  ;
%             sin(-theta)-2*q(2)*q(4)-2*q(1)*q(3);
%             tan(psi)-(2*q(2)*q(3)-2*q(1)*q(4))/(2*q(1)^2+2*q(2)^2-1);
%             q(1)^2+q(2)^2+q(3)^2+q(4)^2-1];
%     end  % Este algoritmo da q* !!!!!

q=[ cos(psi/2)*cos(theta/2)*cos(phi/2)+ sin(psi/2)*sin(theta/2)*sin(phi/2) ;
      cos(psi/2)*cos(theta/2)*sin(phi/2)- sin(psi/2)*sin(theta/2)*cos(phi/2) ;
       cos(psi/2)*sin(theta/2)*cos(phi/2)+ sin(psi/2)*cos(theta/2)*sin(phi/2)   ;
        sin(psi/2)*cos(theta/2)*cos(phi/2)- cos(psi/2)*sin(theta/2)*sin(phi/2)      ]; % Esto nos da q !!!

    function Product= HamiltonProduct( a,b )

Product=[ a(1)*b(1)-a(2)*b(2)-a(3)*b(3)-a(4)*b(4) ; a(1)*b(2)+a(2)*b(1)+a(3)*b(4)-a(4)*b(3)  ; a(1)*b(3)-a(2)*b(4)+a(3)*b(1)+a(4)*b(2)  ; a(1)*b(4)+a(2)*b(3)-a(3)*b(2)+a(4)*b(1) ];

== matlab function Tricopter_Controlled/3 Copter Complete/6dof Eqs of motion/SV_F_b_to_SV_FI ==
  data: V_b input; q_dot input; q input; V_e output; euler output; euler_dot output
function [V_e,euler,euler_dot]   = SV_F_b_to_SV_FI(  V_b, q_dot,q)

xp=V_b(1);
yp=V_b(2);
zp=V_b(3);

%% Velocity and position in Earth Frame   q . v . q*

SolProd=HamiltonProduct([q(1);q(2);q(3);q(4)],HamiltonProduct([0;xp;yp;zp],[q(1);-q(2);-q(3);-q(4)]) );
V_e=SolProd(2:4);

%% Actitud en Angulos de Euler y sus derivadas. 
euler=[0,0,0]';
euler(1,1) = atan2(2*q(3)*q(4)+2*q(1)*q(2),2*q(1)^2+2*q(4)^2-1 ); % phi
euler(2,1) = -asin( 2*q(2)*q(4)-2*q(1)*q(3) ); %  theta
euler(3,1) = atan2( 2*q(2)*q(3)+2*q(1)*q(4),2*q(1)^2+2*q(2)^2-1 ); %  psi

euler_dot=[0,0,0]';
euler_dot(1,1) = 2/(1+( (2*q(3)*q(4)+2*q(1)*q(2))/(2*q(1)^2+2*q(4)^2-1)  )^2)*[ -(2*q(1)^2*q(2)+ 4*q(1)*q(3)*q(4)-2*q(2)*q(4)^2+q(2))  ,  q(1)*(2*q(1)^2+2*q(4)^2-1)  ,  q(4)*(2*q(1)^2+2*q(4)^2-1)  ,  -(-2*q(1)^2*q(3) +4*q(1)*q(2)*q(4)+2*q(3)*q(4)^2+q(3) ) ]*q_dot.* 1/(2*q(1)^2+2*q(4)^2-1)^2; % Derivada de phi
euler_dot(2,1) = -2/( sqrt(1-4*(q(2)*q(4)-q(1)*q(3))^2)  )*[-q(3),q(4),-q(1),q(2)]*q_dot;  % Theta prima
euler_dot(3,1) = 2/(1+( (2*q(2)*q(3)+2*q(1)*q(4))/(2*q(1)^2+2*q(2)^2-1)  )^2)*[  -(2*q(1)^2*q(4)+4*q(1)*q(2)*q(3)-2*q(2)^2*q(4)+q(4)  ) , 1/2*(q(3)*(4*q(1)^2-4*q(2)^2-2)-8*q(1)*q(2)*q(4) )  ,  q(2)*(2*q(1)^2+2*q(2)^2-1)  , q(1)*(2*q(1)^2+2*q(2)^2-1) ]*q_dot.*1/(2*q(1)^2+2*q(2)^2-1)^2;  % Psi prima


function Product= HamiltonProduct( a,b )

Product=[ a(1)*b(1)-a(2)*b(2)-a(3)*b(3)-a(4)*b(4) ; a(1)*b(2)+a(2)*b(1)+a(3)*b(4)-a(4)*b(3)  ; a(1)*b(3)-a(2)*b(4)+a(3)*b(1)+a(4)*b(2)  ; a(1)*b(4)+a(2)*b(3)-a(3)*b(2)+a(4)*b(1) ];

== matlab function Tricopter_Controlled/3 Copter Complete/Mass Properties/Arm Inertia ==
  data: T1_FAFb input; T2_FAFb input; T3_FAFb input; I_M output; l parameter; h_M parameter; m_M parameter; r1_M output; r2_M output; r3_M output
function [I_M,r1_M,r2_M,r3_M]  = Arm1_inertia(T1_FAFb,T2_FAFb,T3_FAFb, l, h_M, m_M)


r1_M=[l;0;0]+T1_FAFb*[0;0;-h_M];
r2_M=[-1/2*l;sqrt(3)/2*l;0]+T2_FAFb*[0;0;-h_M];
r3_M=[-1/2*l;-sqrt(3)/2*l;0]+T3_FAFb*[0;0;-h_M];


I_M1 = m_M*[ r1_M(2)^2+r1_M(3)^2,r1_M(1)*r1_M(2),r1_M(1)*r1_M(3);...
            r1_M(1)*r1_M(2), r1_M(1)^2+r1_M(3)^2, r1_M(2)*r1_M(3);...
            r1_M(1)*r1_M(3),r1_M(2)*r1_M(3), r1_M(1)^2+r1_M(2)^2];
I_M2 = m_M*[ r2_M(2)^2+r2_M(3)^2,r2_M(1)*r2_M(2),r2_M(1)*r2_M(3);...
            r2_M(1)*r2_M(2), r2_M(1)^2+r2_M(3)^2, r2_M(2)*r2_M(3);...
            r2_M(1)*r2_M(3),r2_M(2)*r2_M(3), r2_M(1)^2+r2_M(2)^2];
I_M3 = m_M*[ r3_M(2)^2+r3_M(3)^2,r3_M(1)*r3_M(2),r3_M(1)*r3_M(3);...
            r3_M(1)*r3_M(2), r3_M(1)^2+r3_M(3)^2, r3_M(2)*r3_M(3);...
            r3_M(1)*r3_M(3),r3_M(2)*r3_M(3), r3_M(1)^2+r3_M(2)^2];

I_M = I_M1+I_M2+I_M3;

== matlab function Tricopter_Controlled/TriCopter FCS/TriCopter FCS/Control and guidance/NDI/3Copter_4_NDI&CA/Mass Properties/Arm Inertia ==
  data: T1_FAFb input; T2_FAFb input; T3_FAFb input; I_M output; l parameter; h_M parameter; m_M parameter; r1_M output; r2_M output; r3_M output
function [I_M,r1_M,r2_M,r3_M]  = Motor_steiner(T1_FAFb,T2_FAFb,T3_FAFb, l, h_M, m_M)


r1_M=[l;0;0]+T1_FAFb*[0;0;-h_M];
r2_M=[-1/2*l;sqrt(3)/2*l;0]+T2_FAFb*[0;0;-h_M];
r3_M=[-1/2*l;-sqrt(3)/2*l;0]+T3_FAFb*[0;0;-h_M];


I_M1 = m_M*[ r1_M(2)^2+r1_M(3)^2,r1_M(1)*r1_M(2),r1_M(1)*r1_M(3);...
            r1_M(1)*r1_M(2), r1_M(1)^2+r1_M(3)^2, r1_M(2)*r1_M(3);...
            r1_M(1)*r1_M(3),r1_M(2)*r1_M(3), r1_M(1)^2+r1_M(2)^2];
I_M2 = m_M*[ r2_M(2)^2+r2_M(3)^2,r2_M(1)*r2_M(2),r2_M(1)*r2_M(3);...
            r2_M(1)*r2_M(2), r2_M(1)^2+r2_M(3)^2, r2_M(2)*r2_M(3);...
            r2_M(1)*r2_M(3),r2_M(2)*r2_M(3), r2_M(1)^2+r2_M(2)^2];
I_M3 = m_M*[ r3_M(2)^2+r3_M(3)^2,r3_M(1)*r3_M(2),r3_M(1)*r3_M(3);...
            r3_M(1)*r3_M(2), r3_M(1)^2+r3_M(3)^2, r3_M(2)*r3_M(3);...
            r3_M(1)*r3_M(3),r3_M(2)*r3_M(3), r3_M(1)^2+r3_M(2)^2];

I_M = I_M1+I_M2+I_M3;

== matlab function Tricopter_Controlled/TriCopter FCS/TriCopter FCS/Control and guidance/NDI/3Copter_4_NDI&CA/Perturbations ==
  data: epsilon input; Ctrl_input input; Pert_Ctrl output
function Pert_Ctrl  = Perturbate_input(epsilon, Ctrl_input)
% The control input has a dimension of 9
% The gradient is computed with 2 evaluations, so the output vector has
% 2*9*9 variables

Pert_Ctrl=zeros(2*9*9,1);

for i=1:9
    % Left
    tmp=Ctrl_input;
    tmp(i)=tmp(i)-epsilon;
    Pert_Ctrl( 1+2*(i-1)*9:(2*i-1)*9 ) = tmp;
    % Right
    tmp=Ctrl_input;
    tmp(i)=tmp(i)+epsilon;
    Pert_Ctrl( 1+(2*i-1)*9 :2*i*9 ) = tmp;
end






end

== matlab function Tricopter_Controlled/TriCopter FCS/TriCopter FCS/Flight mode manager and commands generator/Flight manager/flight_mode_manager ==
  data: flight_mode_reqest input; Safety_stab_switch input; flight_mode_out output; p_dop input; num_sats input; Xe input; Vyaw input; Euler input; Volt input; flight_mode input; NOT_allowed_sign output
function [flight_mode_out,NOT_allowed_sign]   =  flight_mode_manager(flight_mode_reqest,Safety_stab_switch,p_dop,num_sats,Xe,Vyaw,Euler,Volt,flight_mode)
% Include here not allowed transitions of flight modes!!

%% monitor stab switch
if Safety_stab_switch==1
    flight_mode_reqest=6;
end

%% CHANGE ALTITUDE FOR WORKING ONLY WITH POSITIVE VALUES
Xe(3)=-Xe(3);


%% By default:
flight_mode_out = flight_mode; % Unless allowed change
NOT_allowed_sign = 0;

%% Allowed transitions logic
if flight_mode_reqest~=flight_mode
    switch flight_mode % Being in this FM
        case 0 % Off
            if flight_mode_reqest==1 && (num_sats>=4 && p_dop<2.5 && Volt > 14.0 && abs(Euler(1))<0.1 && abs(Euler(2))<0.1 )
                flight_mode_out = flight_mode_reqest;
            end
        case 1 % Ready
            if flight_mode_reqest==0
                flight_mode_out = flight_mode_reqest;
            end
            if flight_mode_reqest==2 && (num_sats>=4 && p_dop<2.5 && Volt > 14.0 && abs(Euler(1))<0.1 && abs(Euler(2))<0.1 ) % Add take off configuration
                flight_mode_out = flight_mode_reqest;
            end
        case 2 % Take off
            if (flight_mode_reqest==6 || flight_mode_reqest==7 || flight_mode_reqest==8 || flight_mode_reqest==9)
                flight_mode_out = flight_mode_reqest;
            end
            if (flight_mode_reqest==3 || flight_mode_reqest==4 || flight_mode_reqest==5) && (num_sats>=4 && p_dop<2.5 && abs(Euler(1))<0.1 && abs(Euler(2))<0.1 && Xe(3)>0.3 )
                flight_mode_out = flight_mode_reqest;
            end
            
        case 3 % Full_auto
            if (flight_mode_reqest==6 || flight_mode_reqest==7 || flight_mode_reqest==8 || flight_mode_reqest==9)
                flight_mode_out = flight_mode_reqest;
            end
            if ( flight_mode_reqest==4 || flight_mode_reqest==5) && (num_sats>=4 && p_dop<2.5 && abs(Euler(1))<0.1 && abs(Euler(2))<0.1 && Xe(3)>0.3 )
                flight_mode_out = flight_mode_reqest;
            end
        case 4 % Vel_height_auto
            if (flight_mode_reqest==6 || flight_mode_reqest==7 || flight_mode_reqest==8 || flight_mode_reqest==9)
                flight_mode_out = flight_mode_reqest;
            end
            if (flight_mode_reqest==3 || flight_mode_reqest==5) && (num_sats>=4 && p_dop<2.5 && abs(Euler(1))<0.1 && abs(Euler(2))<0.1 && Xe(3)>0.3 )
                flight_mode_out = flight_mode_reqest;
            end
        case 5 % Vel_auto
            if (flight_mode_reqest==6 || flight_mode_reqest==7 || flight_mode_reqest==8 || flight_mode_reqest==9)
                flight_mode_out = flight_mode_reqest;
            end
            if (flight_mode_reqest==3 || flight_mode_reqest==4 ) && (num_sats>=4 && p_dop<2.5 && abs(Euler(1))<0.1 && abs(Euler(2))<0.1 && Xe(3)>0.3 )
                flight_mode_out = flight_mode_reqest;
            end
        case 6 % Stab
            if ( flight_mode_reqest==7 || flight_mode_reqest==8 || flight_mode_reqest==9)
                flight_mode_out = flight_mode_reqest;
            end
            if (flight_mode_reqest==3 || flight_mode_reqest==4 || flight_mode_reqest==5) && (num_sats>=4 && p_dop<2.5 && abs(Euler(1))<0.1 && abs(Euler(2))<0.1 && Xe(3)>0.3 )
                flight_mode_out = flight_mode_reqest;
            end
        case 7 % Man_ctrl
            if (flight_mode_reqest==6 || flight_mode_reqest==8 || flight_mode_reqest==9)
                flight_mode_out = flight_mode_reqest;
            end
            if (flight_mode_reqest==3 || flight_mode_reqest==4 || flight_mode_reqest==5) && (num_sats>=4 && p_dop<2.5 && abs(Euler(1))<0.1 && abs(Euler(2))<0.1 && Xe(3)>0.3 )
                flight_mode_out = flight_mode_reqest;
            end
        case 8 % Home
            if (flight_mode_reqest==6 || flight_mode_reqest==7 || flight_mode_reqest==9)
                flight_mode_out = flight_mode_reqest;
            end
            if (flight_mode_reqest==3 || flight_mode_reqest==4 || flight_mode_reqest==5) && (num_sats>=4 && p_dop<2.5 && abs(Euler(1))<0.1 && abs(Euler(2))<0.1 && Xe(3)>0.3 )
                flight_mode_out = flight_mode_reqest;
            end
        case 9 % Land
            if (flight_mode_reqest==1 || flight_mode_reqest==2)
                flight_mode_out = flight_mode_reqest;
            end
        otherwise
            flight_mode_out = flight_mode; % Unless allowed change
            
    end
    

end

% If not allowed change:
if flight_mode_reqest~=flight_mode_out
    NOT_allowed_sign = 1; % Make anything
end

== matlab function Tricopter_Controlled/TriCopter FCS/TriCopter FCS/Px4_to_simulink input interface/MATLAB Function ==
  data: T_yaw output; yaw input
function T_yaw = Yaw_rotate(yaw)


T_yaw=[cos(yaw),    sin(yaw),   0;
        -sin(yaw),  cos(yaw),   0;
        0,      0,              1];

== matlab function Tricopter_Controlled/TriCopter FCS/TriCopter FCS/Flight mode manager and commands generator/Commands generator/commnads_gen_logic/commands_generator ==
  data: flight_mode input; Xe input; V_yaw input; Euler input; Loc_XY_sp output; Alt_sp output; Vel_yaw_xy_sp output; Vel_yaw_z_sp output; att_sp output; omega_b_sp output; K_alt output; K_x output; K_y output; K_vx output; K_vy output; K_vz output; K_phi output; K_theta output; K_yaw output; K_p output; K_q output; K_r output; Ix parameter; Iy parameter; Iz parameter
function [Loc_XY_sp,Alt_sp,Vel_yaw_xy_sp,Vel_yaw_z_sp,att_sp,omega_b_sp , K_alt,K_x,K_y,K_vx,K_vy,K_vz,K_phi,K_theta,K_yaw,K_p,K_q,K_r]  =  commands_generator(flight_mode,Xe,V_yaw,Euler,Ix,Iy,Iz)
%% Generador de comandos (iniciales al menos) para cada fliht_mode



%% Pro precaucion, le damos la vuelta a la altura
Xe(3)=-Xe(3);

switch flight_mode
    case 0 % Off
        Loc_XY_sp       = [0,0]';
        Alt_sp          = 0; 
        Vel_yaw_xy_sp   = [0,0]';
        Vel_yaw_z_sp    = 0;
        att_sp          = [0,0,0]';
        omega_b_sp      = [0,0,0]';
        
        K_alt           = 0;
        K_x             = 0;
        K_y             = 0;
        K_vx            = 0;
        K_vy            = 0;
        K_vz            = 0;
        K_phi            = 0;
        K_theta            = 0;
        K_yaw           = 0;
        K_p            = 0;
        K_q            = 0;
        K_r            = 0;
    case 1 % Ready        
        Loc_XY_sp       = [0,0]';
        Alt_sp          = 0; 
        Vel_yaw_xy_sp   = [0,0]';
        Vel_yaw_z_sp    = 0;
        att_sp          = [0,0,0]';
        omega_b_sp      = [0,0,0]';

        K_alt           = 0;
        K_x             = 0;
        K_y             = 0;
        K_vx            = 0;
        K_vy            = 0;
        K_vz            = 0;
        K_phi           = 0;
        K_theta         = 0;
        K_yaw           = 0;

        K_p            = 0;
        K_q            = 0;
        K_r            = 0;
    case 2 % Take off
        Loc_XY_sp       = [0,0]';
        Alt_sp          = 1; 
        Vel_yaw_xy_sp   = [0,0]';
        Vel_yaw_z_sp    = 0;
        att_sp          = [0,0,Euler(3)]';
        omega_b_sp      = [0,0,0]';

        K_alt           = 1;
        K_x             = 0;
        K_y             = 0;
        K_vx            = 0;
        K_vy            = 0;
        K_vz            = 0;
        K_phi           = 0;
        K_theta        = 0;
        K_yaw           = 0;

        K_p            = 0;
        K_q            = 0;
        K_r            = 0;
    case 3 % Full_auto
        Loc_XY_sp       = [Xe(1),Xe(2)]';
        Alt_sp          = Xe(3); 
        Vel_yaw_xy_sp   = [0,0]';
        Vel_yaw_z_sp    = 0;
        att_sp          = [0,0,Euler(3)]';
        omega_b_sp      = [0,0,0]';

        K_alt           = 1;
        K_x             = 1;
        K_y             = 1;
        K_vx            = 0;
        K_vy            = 0;
        K_vz            = 0;
        K_phi            = 0;
        K_theta            = 0;
        K_yaw           = pi/180*(90);
        K_p            = 0;
        K_q            = 0;
        K_r            = 0;
    case 4 % Vel_height_auto
        Loc_XY_sp       = [0,0]';
        Alt_sp          = Xe(3); 
        Vel_yaw_xy_sp   = [0,0]';
        Vel_yaw_z_sp    = 0;
        att_sp          = [0,0,Euler(3)]';
        omega_b_sp      = [0,0,0]';

        K_alt           = 1;
        K_x             = 0;
        K_y             = 0;
        K_vx            = 1;
        K_vy            = 1;
        K_vz            = 0;
        K_phi            = 0;
        K_theta            = 0;
        K_yaw           = pi/180*(90);
        K_p            = 0;
        K_q            = 0;
        K_r            = 0;
    case 5 % Vel_auto
        Loc_XY_sp       = [0,0]';
        Alt_sp          = 0; 
        Vel_yaw_xy_sp   = [0,0]';
        Vel_yaw_z_sp    = 0;
        att_sp          = [0,0,Euler(3)]';
        omega_b_sp      = [0,0,0]';

        K_alt           = 0;
        K_x             = 0;
        K_y             = 0;
        K_vx            = 1;
        K_vy            = 1;
        K_vz            = 1;
        K_phi           = 0;
        K_theta         = 0;
        K_yaw           = pi/180*(90);
        K_p            = 0;
        K_q            = 0;
        K_r            = 0;
    case 6 % Stab
        Loc_XY_sp       = [0,0]';
        Alt_sp          = 0; 
        Vel_yaw_xy_sp   = [0,0]';
        Vel_yaw_z_sp    = 0;
        att_sp          = [0,0,Euler(3)]';
        omega_b_sp      = [0,0,0]';

        K_alt           = 0;
        K_x             = 0;
        K_y             = 0;
        K_vx            = 0;
        K_vy            = 0;
        K_vz            = 1;
        K_phi           = pi/180*10;
        K_theta         = pi/180*10;
        K_yaw           = pi/180*(90);
        K_p            = 0;
        K_q            = 0;
        K_r            = 0;
    case 7 % Man_ctrl
        Loc_XY_sp       = [0,0]';
        Alt_sp          = 0; 
        Vel_yaw_xy_sp   = [0,0]';
        Vel_yaw_z_sp    = 0;
        att_sp          = [0,0,0]';
        omega_b_sp      = [0,0,0]';

        K_alt           = 0;
        K_x             = 0;
        K_y             = 0;
        K_vx            = 0;
        K_vy            = 0;
        K_vz            = 1;
        K_phi           = 0;
        K_theta         = 0;
        K_yaw           = 0;
        K_p            = pi/180*(2);
        K_q            = pi/180*(2);
        K_r            = pi/180*(2);
    case 8 % Home
        Loc_XY_sp       = [0,0]';
        Alt_sp          = 0.5; 
        Vel_yaw_xy_sp   = [0,0]';
        Vel_yaw_z_sp    = 0;
        att_sp          = [0,0,Euler(3)]';
        omega_b_sp      = [0,0,0]';

        K_alt           = 0;
        K_x             = 0;
        K_y             = 0;
        K_vx            = 0;
        K_vy            = 0;
        K_vz            = 0;
        K_phi            = 0;
        K_theta            = 0;
        K_yaw           = 0;
        K_p            = 0;
        K_q            = 0;
        K_r            = 0;
    case 9 % Land
        Loc_XY_sp       = [Xe(1),Xe(2)]';
        Alt_sp          = 0; 
        Vel_yaw_xy_sp   = [0,0]';
        Vel_yaw_z_sp    = 0;
        att_sp          = [0,0,Euler(3)]';
        omega_b_sp      = [0,0,0]';

        K_alt           = 0;
        K_x             = 0;
        K_y             = 0;
        K_vx            = 0;
        K_vy            = 0;
        K_vz            = 0;
        K_phi            = 0;
        K_theta            = 0;
        K_yaw           = 0;
        K_p            = 0;
        K_q            = 0;
        K_r            = 0;
    otherwise
        Loc_XY_sp       = [0,0]';
        Alt_sp          = 0; 
        Vel_yaw_xy_sp   = [0,0]';
        Vel_yaw_z_sp    = 0;
        att_sp          = [0,0,Euler(3)]';
        omega_b_sp      = [0,0,0]';

        K_alt           = 0;
        K_x             = 0;
        K_y             = 0;
        K_vx            = 0;
        K_vy            = 0;
        K_vz            = 0;
        K_phi            = 0;
        K_theta            = 0;
        K_yaw           = 0;
        K_p            = 0;
        K_q            = 0;
        K_r            = 0;
end
